simulink model "PE_V2_0"  (R2020b)
settings: Solver=VariableStepAuto  StartTime=0.0  StopTime=10.0  RelTol=1e-3
undefined symbols (not defined in the file): ZERO
libraries: hdlsllib x35, simulink x28, visionhdlutilities x12
(part 2 of 3)

== system PE_V2_0/2DConvPE1 V2.0/Subsystem2 ==
  In1 : Inport
  Bus Selector : BusSelector  OutputSignals=signal1,signal2,signal3,signal4,signal5,signal6,signal7,signal8,signal9,signal10,signal11,signal12,signal13,signal14,signal15
  Weight_Length : Outport
  Weight_Area : Outport  Port=2
  Weight_Width : Outport  Port=3
  Weight_Height : Outport  Port=4
  Feature_Length : Outport  Port=5
  Feature_Area : Outport  Port=6
  Feature_Width : Outport  Port=7
  Feature_Height : Outport  Port=8
  outFeature_Length : Outport  Port=9
  outFeature_Area : Outport  Port=10
  outFeature_Width : Outport  Port=11
  outFeature_Height : Outport  Port=12
  Conv_Step : Outport  Port=13
  Phase_in : Outport  Port=14
  Phase_out : Outport  Port=15
  wires:
  In1/1 -> Bus Selector/1
  Bus Selector/1 -> Weight_Length/1  "<signal1>"
  Bus Selector/2 -> Weight_Area/1  "<signal2>"
  Bus Selector/3 -> Weight_Width/1  "<signal3>"
  Bus Selector/4 -> Weight_Height/1  "<signal4>"
  Bus Selector/5 -> Feature_Length/1  "<signal5>"
  Bus Selector/6 -> Feature_Area/1  "<signal6>"
  Bus Selector/7 -> Feature_Width/1  "<signal7>"
  Bus Selector/8 -> Feature_Height/1  "<signal8>"
  Bus Selector/9 -> outFeature_Length/1  "<signal9>"
  Bus Selector/10 -> outFeature_Area/1  "<signal10>"
  Bus Selector/11 -> outFeature_Width/1  "<signal11>"
  Bus Selector/12 -> outFeature_Height/1  "<signal12>"
  Bus Selector/13 -> Conv_Step/1  "<signal13>"
  Bus Selector/14 -> Phase_in/1  "<signal14>"
  Bus Selector/15 -> Phase_out/1  "<signal15>"

== system PE_V2_0/2DCov PEV1.1/Adder Tree ==
  In1 : Inport
  In2 : Inport  Port=2
  In3 : Inport  Port=3
  In4 : Inport  Port=4
  In5 : Inport  Port=5
  In6 : Inport  Port=6
  In7 : Inport  Port=7
  In8 : Inport  Port=8
  In9 : Inport  Port=9
  validIn : Inport  Port=10
  Add{,1..6,10} (8 alike) : Sum
  Delay{1..9,35} (10 alike) : Delay  DelayLength=1
  Out1 : Outport
  validOut : Outport  Port=2
  wires:
  Add/1 -> Add4/1
  Add4/1 -> Add6/1
  Add10/1 -> Out1/1
  Add3/1 -> Add5/2
  Add2/1 -> Add5/1
  Add1/1 -> Add4/2
  Add6/1 -> Add10/1
  Add5/1 -> Add6/2
  Delay35/1 -> Add/1
  Delay1/1 -> Add/2
  Delay3/1 -> Add1/1
  Delay2/1 -> Add1/2
  Delay5/1 -> Add2/1
  Delay4/1 -> Add2/2
  Delay7/1 -> Add3/1
  Delay6/1 -> Add3/2
  In9/1 -> Delay8/1
  Delay8/1 -> Add10/2
  In8/1 -> Delay6/1
  In7/1 -> Delay7/1
  In6/1 -> Delay4/1
  In5/1 -> Delay5/1
  In4/1 -> Delay2/1
  In3/1 -> Delay3/1
  In2/1 -> Delay1/1
  In1/1 -> Delay35/1
  validIn/1 -> Delay9/1
  Delay9/1 -> validOut/1

== system PE_V2_0/2DCov PEV1.1/Address Logic ==
  note: W/R_Address_Gen
  In1 : Inport
  In2 : Inport  Port=2
  " " : Subsystem
  Add : Sum  Inputs=+-
  Compare To Constant : simulink/Logic and Bit Operations/Compare To Constant  relop===  const=0  OutDataTypeStr=boolean
  Constant : Constant  OutDataTypeStr=uint32
  Delay : Delay  DelayLength=1
  Logical Operator1 : Logic  AllPortsSameDT=off  OutDataTypeStr=boolean
  Logical Operator2 : Logic  Operator=NOT  AllPortsSameDT=off  OutDataTypeStr=boolean
  Relational Operator : RelationalOperator  OutDataTypeStr=boolean  RndMeth=Simplest
  Weight_Counter : hdlsllib/Sources/HDL Counter  CountType=Free running  CountInit=0  CountStep=1  CountMax=2^15  CountFromType=Initial value  CountFrom=0  CountResetPort=on  CountLoadPort=off  CountEnbPort=on  CountDirPort=off  CountDataType=Unsigned  CountWordLen=32  CountFracLen=0  CountSampTime=1
  Weight_Interation_Counter : hdlsllib/Sources/HDL Counter  CountType=Free running  CountInit=0  CountStep=1  CountMax=2^15  CountFromType=Initial value  CountFrom=0  CountResetPort=on  CountLoadPort=off  CountEnbPort=on  CountDirPort=off  CountDataType=Unsigned  CountWordLen=32  CountFracLen=0  CountSampTime=1
  W : Outport
  Write_en : Outport  Port=2
  R : Outport  Port=3
  wires:
  Weight_Counter/1 -> " "/1(In1), Relational Operator/1
  Compare To Constant/1 -> Write_en/1, " "/2(In2)
  Delay/1 -> Logical Operator1/2, Logical Operator2/1, Weight_Counter/2
  Weight_Interation_Counter/1 -> Compare To Constant/1
  Constant/1 -> Add/2
  Logical Operator2/1 -> Weight_Interation_Counter/1
  " "/1(W) -> W/1
  Logical Operator1/1 -> Weight_Counter/1
  Relational Operator/1 -> Weight_Interation_Counter/2, Logical Operator1/1
  Add/1 -> Relational Operator/2
  In1/1 -> Delay/1
  In2/1 -> Add/1
  " "/2(R) -> R/1

== system PE_V2_0/2DCov PEV1.1/LIne Buffer ==
  Stream_In : Inport
  Stream_Valid : Inport  Port=2
  Weight_Width : Inport  Port=3
  Feature_Area : Inport  Port=4
  Feature_Width : Inport  Port=5
  Feature_Height : Inport  Port=6
  Delay2 : Delay  DelayLength=1
  Line Buffer : Subsystem
  OutValidGen : Subsystem
  Terminator : Terminator
  pixel : Outport
  valid : Outport  Port=2
  wires:
  Feature_Area/1 -> Line Buffer/3(Feature_Area)
  Feature_Height/1 -> OutValidGen/3(Feature_Height)
  Line Buffer/3(shftEnable) -> Terminator/1
  Stream_In/1 -> Line Buffer/1(Stream_In)
  Line Buffer/1(pixel) -> Delay2/1
  Line Buffer/2(ctrl) -> OutValidGen/1(In1)
  Feature_Width/1 -> Line Buffer/4(Feature_Width)
  Stream_Valid/1 -> Line Buffer/2(Stream_Valid)
  Weight_Width/1 -> OutValidGen/2(Weight_Width)
  OutValidGen/1(valid) -> valid/1
  Delay2/1 -> pixel/1

== system PE_V2_0/2DCov PEV1.1/MaxPooling ==
  Stream_In : Inport
  Stream_Valid : Inport  Port=2
  ByPass : Inport  Port=3
  step : Inport  Port=4
  Window_Width : Inport  Port=5
  Feature_Area : Inport  Port=6
  Feature_Width : Inport  Port=7
  Feature_Height : Inport  Port=8
  Comparator : Subsystem
  Constant : Constant  Value=0  OutDataTypeStr=int32
  Delay{,1..6,36} (8 alike) : Delay  DelayLength=1
  Line Buffer1 : Subsystem
  OutValidGen : Subsystem
  Switch : Switch  Criteria=u2 > Threshold
  Switch1 : Switch  Criteria=u2 > Threshold
  Terminator1 : Terminator
  dataSwitch : Switch  Criteria=u2 > Threshold
  validSwitch : Switch  Criteria=u2 > Threshold
  window Selector : Subsystem
  outdata : Outport
  Valid : Outport  Port=2
  wires:
  window Selector/3(Out3) -> Delay3/1
  OutValidGen/1(Out1) -> window Selector/2(valid)
  Feature_Width/1 -> Line Buffer1/4(Feature_Width)
  Line Buffer1/3(shftEnable) -> Terminator1/1
  Window_Width/1 -> OutValidGen/2(Window_Width)
  window Selector/5(Valid) -> Delay5/1
  window Selector/1(Out1) -> Delay/1
  Line Buffer1/1(pixel) -> Delay2/1
  Line Buffer1/2(ctrl) -> OutValidGen/1(ctrl)
  window Selector/2(Out2) -> Delay6/1
  window Selector/4(Out4) -> Delay4/1
  Feature_Area/1 -> Line Buffer1/3(Feature_Area)
  Feature_Height/1 -> OutValidGen/3(Feature_Height)
  step/1 -> window Selector/3(step)
  Delay1/1 -> validSwitch/1, Switch1/3
  Comparator/1(Out1) -> dataSwitch/3
  Delay36/1 -> dataSwitch/1, Switch/3
  ByPass/1 -> validSwitch/2, dataSwitch/2, Switch1/2, Switch/2
  dataSwitch/1 -> outdata/1
  validSwitch/1 -> Valid/1
  Constant/1 -> Switch1/1, Switch/1
  Switch/1 -> Line Buffer1/1(Stream_In)
  Switch1/1 -> Line Buffer1/2(Stream_Valid)
  Comparator/2(outvalid) -> validSwitch/3
  Stream_In/1 -> Delay36/1
  Stream_Valid/1 -> Delay1/1
  Delay2/1 -> window Selector/1(pixel)
  Delay/1 -> Comparator/1(In1)
  Delay5/1 -> Comparator/5(Valid)
  Delay4/1 -> Comparator/4(In4)
  Delay3/1 -> Comparator/3(In3)
  Delay6/1 -> Comparator/2(In2)

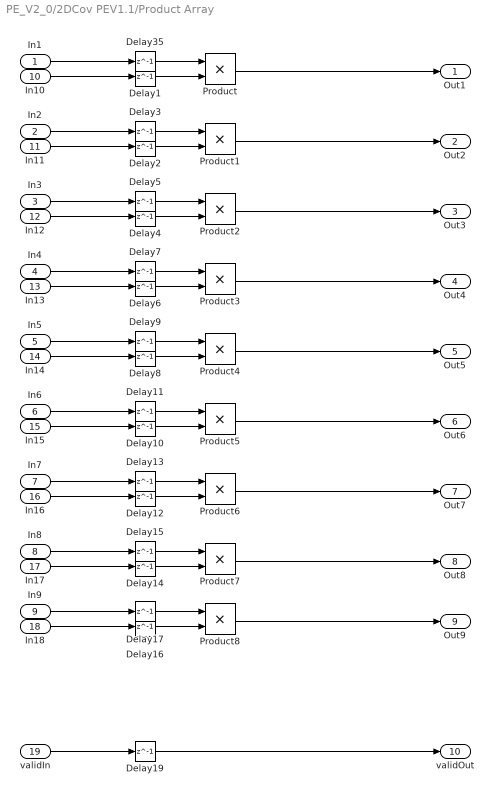
== system PE_V2_0/2DCov PEV1.1/Product Array ==
  In1 : Inport
  In2 : Inport  Port=2
  In3 : Inport  Port=3
  In4 : Inport  Port=4
  In5 : Inport  Port=5
  In6 : Inport  Port=6
  In7 : Inport  Port=7
  In8 : Inport  Port=8
  In9 : Inport  Port=9
  In10 : Inport  Port=10
  In11 : Inport  Port=11
  In12 : Inport  Port=12
  In13 : Inport  Port=13
  In14 : Inport  Port=14
  In15 : Inport  Port=15
  In16 : Inport  Port=16
  In17 : Inport  Port=17
  In18 : Inport  Port=18
  validIn : Inport  Port=19
  Delay{1..17,19,35} (19 alike) : Delay  DelayLength=1
  Product{,1..8} (9 alike) : Product
  Out1 : Outport
  Out2 : Outport  Port=2
  Out3 : Outport  Port=3
  Out4 : Outport  Port=4
  Out5 : Outport  Port=5
  Out6 : Outport  Port=6
  Out7 : Outport  Port=7
  Out8 : Outport  Port=8
  Out9 : Outport  Port=9
  validOut : Outport  Port=10
  wires:
  Product/1 -> Out1/1
  In4/1 -> Delay7/1
  Product4/1 -> Out5/1
  In8/1 -> Delay15/1
  In17/1 -> Delay14/1
  In9/1 -> Delay17/1
  In12/1 -> Delay4/1
  In7/1 -> Delay13/1
  In1/1 -> Delay35/1
  In13/1 -> Delay6/1
  Product1/1 -> Out2/1
  In16/1 -> Delay12/1
  In10/1 -> Delay1/1
  In14/1 -> Delay8/1
  In18/1 -> Delay16/1
  Product8/1 -> Out9/1
  Product7/1 -> Out8/1
  In6/1 -> Delay11/1
  In2/1 -> Delay3/1
  In11/1 -> Delay2/1
  In15/1 -> Delay10/1
  In5/1 -> Delay9/1
  In3/1 -> Delay5/1
  Product3/1 -> Out4/1
  Product2/1 -> Out3/1
  Product5/1 -> Out6/1
  Product6/1 -> Out7/1
  validIn/1 -> Delay19/1
  Delay1/1 -> Product/2
  Delay35/1 -> Product/1
  Delay3/1 -> Product1/1
  Delay2/1 -> Product1/2
  Delay5/1 -> Product2/1
  Delay4/1 -> Product2/2
  Delay7/1 -> Product3/1
  Delay6/1 -> Product3/2
  Delay8/1 -> Product4/2
  Delay9/1 -> Product4/1
  Delay11/1 -> Product5/1
  Delay10/1 -> Product5/2
  Delay13/1 -> Product6/1
  Delay12/1 -> Product6/2
  Delay14/1 -> Product7/2
  Delay15/1 -> Product7/1
  Delay17/1 -> Product8/1
  Delay16/1 -> Product8/2
  Delay19/1 -> validOut/1

== system PE_V2_0/2DCov PEV1.1/ReLU ==
  data_in : Inport
  validIn : Inport  Port=2
  byPass : Inport  Port=3
  Compare To Zero : simulink/Logic and Bit Operations/Compare To Zero  relop=>  OutDataTypeStr=boolean
  Constant : Constant  Value=0  OutDataTypeStr=int32
  Delay1 : Delay  DelayLength=1
  Delay36 : Delay  DelayLength=1
  Switch : Switch  Criteria=u2 > Threshold
  Switch1 : Switch  Criteria=u2 > Threshold
  data_ReLU : Outport
  valildOut : Outport  Port=2
  wires:
  Constant/1 -> Switch/3
  Delay36/1 -> Switch1/1, Switch/1, Compare To Zero/1
  Compare To Zero/1 -> Switch/2
  Switch/1 -> Switch1/3
  byPass/1 -> Switch1/2
  Switch1/1 -> data_ReLU/1
  Delay1/1 -> valildOut/1
  data_in/1 -> Delay36/1
  validIn/1 -> Delay1/1

== system PE_V2_0/2DCov PEV1.1/Subsystem ==
  In1 : Inport
  Bus Selector : BusSelector  OutputSignals=signal1,signal2
  pool_step : Outport
  pool_Width : Outport  Port=2
  wires:
  Bus Selector/2 -> pool_Width/1  "<signal2>"
  Bus Selector/1 -> pool_step/1  "<signal1>"
  In1/1 -> Bus Selector/1

== system PE_V2_0/2DCov PEV1.1/Subsystem2 ==
  In1 : Inport
  Bus Selector : BusSelector  OutputSignals=signal1,signal2,signal3,signal4,signal5,signal6,signal7,signal8,signal9,signal10,signal11,signal12,signal13,signal14,signal15
  Weight_Length : Outport
  Weight_Area : Outport  Port=2
  Weight_Width : Outport  Port=3
  Weight_Height : Outport  Port=4
  Feature_Length : Outport  Port=5
  Feature_Area : Outport  Port=6
  Feature_Width : Outport  Port=7
  Feature_Height : Outport  Port=8
  outFeature_Length : Outport  Port=9
  outFeature_Area : Outport  Port=10
  outFeature_Width : Outport  Port=11
  outFeature_Height : Outport  Port=12
  Conv_Step : Outport  Port=13
  inChannel : Outport  Port=14
  outChannel : Outport  Port=15
  wires:
  In1/1 -> Bus Selector/1
  Bus Selector/1 -> Weight_Length/1  "<signal1>"
  Bus Selector/2 -> Weight_Area/1  "<signal2>"
  Bus Selector/3 -> Weight_Width/1  "<signal3>"
  Bus Selector/4 -> Weight_Height/1  "<signal4>"
  Bus Selector/5 -> Feature_Length/1  "<signal5>"
  Bus Selector/6 -> Feature_Area/1  "<signal6>"
  Bus Selector/7 -> Feature_Width/1  "<signal7>"
  Bus Selector/8 -> Feature_Height/1  "<signal8>"
  Bus Selector/9 -> outFeature_Length/1  "<signal9>"
  Bus Selector/10 -> outFeature_Area/1  "<signal10>"
  Bus Selector/11 -> outFeature_Width/1  "<signal11>"
  Bus Selector/12 -> outFeature_Height/1  "<signal12>"
  Bus Selector/13 -> Conv_Step/1  "<signal13>"
  Bus Selector/14 -> inChannel/1  "<signal14>"
  Bus Selector/15 -> outChannel/1  "<signal15>"

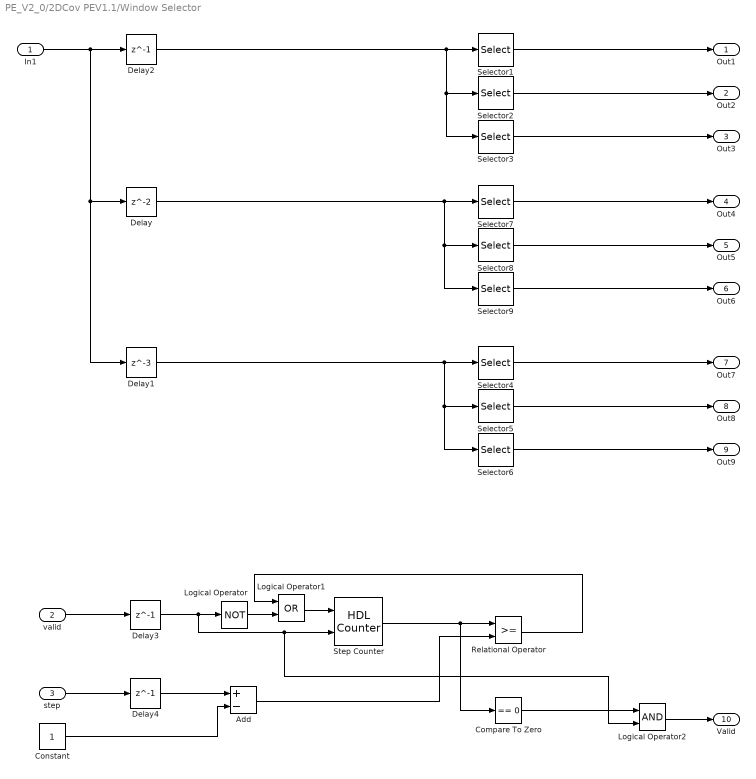
== system PE_V2_0/2DCov PEV1.1/Window Selector ==
  In1 : Inport
  valid : Inport  Port=2
  step : Inport  Port=3
  Add : Sum  Inputs=+-
  Compare To Zero : simulink/Logic and Bit Operations/Compare To Zero  relop===  OutDataTypeStr=boolean
  Constant : Constant  OutDataTypeStr=uint32
  Delay : Delay
  Delay1 : Delay  DelayLength=3
  Delay2 : Delay  DelayLength=1
  Delay3 : Delay  DelayLength=1
  Delay4 : Delay  DelayLength=1
  Logical Operator : Logic  Operator=NOT  AllPortsSameDT=off  OutDataTypeStr=boolean
  Logical Operator1 : Logic  Operator=OR  AllPortsSameDT=off  OutDataTypeStr=boolean
  Logical Operator2 : Logic  AllPortsSameDT=off  OutDataTypeStr=boolean
  Relational Operator : RelationalOperator  OutDataTypeStr=boolean  RndMeth=Nearest
  Selector1 : Selector  InputPortWidth=3  IndexOptions=Index vector (dialog)  Indices=[1]  OutputSizes=1
  Selector2 : Selector  InputPortWidth=3  IndexOptions=Index vector (dialog)  Indices=[2]  OutputSizes=1
  Selector3 : Selector  InputPortWidth=3  IndexOptions=Index vector (dialog)  Indices=[3]  OutputSizes=1
  Selector4 : Selector  InputPortWidth=3  IndexOptions=Index vector (dialog)  Indices=[1]  OutputSizes=1
  Selector5 : Selector  InputPortWidth=3  IndexOptions=Index vector (dialog)  Indices=[2]  OutputSizes=1
  Selector6 : Selector  InputPortWidth=3  IndexOptions=Index vector (dialog)  Indices=[3]  OutputSizes=1
  Selector7 : Selector  InputPortWidth=3  IndexOptions=Index vector (dialog)  Indices=[1]  OutputSizes=1
  Selector8 : Selector  InputPortWidth=3  IndexOptions=Index vector (dialog)  Indices=[2]  OutputSizes=1
  Selector9 : Selector  InputPortWidth=3  IndexOptions=Index vector (dialog)  Indices=[3]  OutputSizes=1
  Step Counter : hdlsllib/Sources/HDL Counter  CountType=Free running  CountInit=0  CountStep=1  CountMax=2^15  CountFromType=Initial value  CountFrom=0  CountResetPort=on  CountLoadPort=off  CountEnbPort=on  CountDirPort=off  CountDataType=Unsigned  CountWordLen=32  CountFracLen=0  CountSampTime=1
  Out1 : Outport
  Out2 : Outport  Port=2
  Out3 : Outport  Port=3
  Out4 : Outport  Port=4
  Out5 : Outport  Port=5
  Out6 : Outport  Port=6
  Out7 : Outport  Port=7
  Out8 : Outport  Port=8
  Out9 : Outport  Port=9
  Valid : Outport  Port=10
  wires:
  Selector2/1 -> Out2/1
  In1/1 -> Delay2/1, Delay1/1, Delay/1
  Selector1/1 -> Out1/1
  Selector3/1 -> Out3/1
  Selector8/1 -> Out5/1
  Selector9/1 -> Out6/1
  Selector7/1 -> Out4/1
  Delay/1 -> Selector9/1, Selector8/1, Selector7/1
  Selector5/1 -> Out8/1
  Selector6/1 -> Out9/1
  Selector4/1 -> Out7/1
  Delay1/1 -> Selector6/1, Selector5/1, Selector4/1
  Relational Operator/1 -> Logical Operator1/1
  Constant/1 -> Add/2
  Logical Operator2/1 -> Valid/1
  Compare To Zero/1 -> Logical Operator2/1
  Logical Operator1/1 -> Step Counter/1
  Logical Operator/1 -> Logical Operator1/2
  Delay4/1 -> Add/1
  Step Counter/1 -> Compare To Zero/1, Relational Operator/1
  Delay3/1 -> Logical Operator2/2, Step Counter/2, Logical Operator/1
  Add/1 -> Relational Operator/2
  Delay2/1 -> Selector3/1, Selector2/1, Selector1/1
  valid/1 -> Delay3/1
  step/1 -> Delay4/1

== system PE_V2_0/2DConvPE1 V1.5/FUNCTION/Adder Tree ==
  In1 : Inport
  In2 : Inport  Port=2
  In3 : Inport  Port=3
  In4 : Inport  Port=4
  In5 : Inport  Port=5
  In6 : Inport  Port=6
  In7 : Inport  Port=7
  In8 : Inport  Port=8
  In9 : Inport  Port=9
  validIn : Inport  Port=10
  Add{,1..6,10} (8 alike) : Sum
  Delay{1..9,35} (10 alike) : Delay  DelayLength=1
  dataOut : Outport
  validOut : Outport  Port=2
  wires:
  Add/1 -> Add4/1
  Add4/1 -> Add6/1
  Add10/1 -> dataOut/1
  Add3/1 -> Add5/2
  Add2/1 -> Add5/1
  Add1/1 -> Add4/2
  Add6/1 -> Add10/1
  Add5/1 -> Add6/2
  Delay35/1 -> Add/1
  Delay1/1 -> Add/2
  Delay3/1 -> Add1/1
  Delay2/1 -> Add1/2
  Delay5/1 -> Add2/1
  Delay4/1 -> Add2/2
  Delay7/1 -> Add3/1
  Delay6/1 -> Add3/2
  In9/1 -> Delay8/1
  Delay8/1 -> Add10/2
  In8/1 -> Delay6/1
  In7/1 -> Delay7/1
  In6/1 -> Delay4/1
  In5/1 -> Delay5/1
  In4/1 -> Delay2/1
  In3/1 -> Delay3/1
  In2/1 -> Delay1/1
  In1/1 -> Delay35/1
  validIn/1 -> Delay9/1
  Delay9/1 -> validOut/1

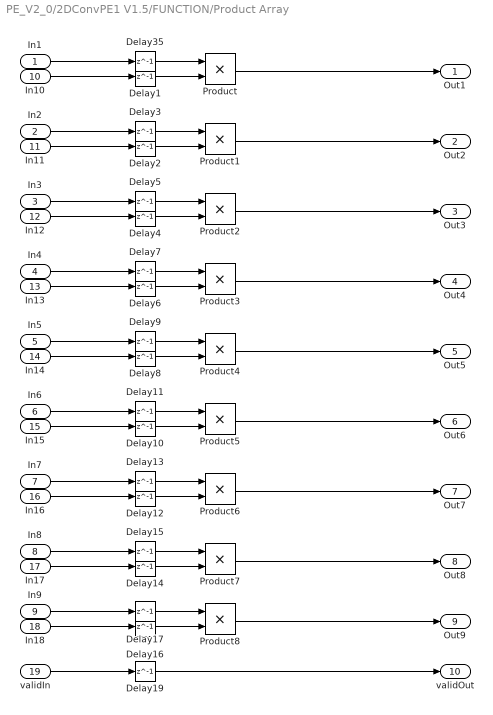
== system PE_V2_0/2DConvPE1 V1.5/FUNCTION/Product Array ==
  In1 : Inport
  In2 : Inport  Port=2
  In3 : Inport  Port=3
  In4 : Inport  Port=4
  In5 : Inport  Port=5
  In6 : Inport  Port=6
  In7 : Inport  Port=7
  In8 : Inport  Port=8
  In9 : Inport  Port=9
  In10 : Inport  Port=10
  In11 : Inport  Port=11
  In12 : Inport  Port=12
  In13 : Inport  Port=13
  In14 : Inport  Port=14
  In15 : Inport  Port=15
  In16 : Inport  Port=16
  In17 : Inport  Port=17
  In18 : Inport  Port=18
  validIn : Inport  Port=19
  Delay{1..17,19,35} (19 alike) : Delay  DelayLength=1
  Product{,1..8} (9 alike) : Product
  Out1 : Outport
  Out2 : Outport  Port=2
  Out3 : Outport  Port=3
  Out4 : Outport  Port=4
  Out5 : Outport  Port=5
  Out6 : Outport  Port=6
  Out7 : Outport  Port=7
  Out8 : Outport  Port=8
  Out9 : Outport  Port=9
  validOut : Outport  Port=10
  wires:
  Product/1 -> Out1/1
  In4/1 -> Delay7/1
  Product4/1 -> Out5/1
  In8/1 -> Delay15/1
  In17/1 -> Delay14/1
  In9/1 -> Delay17/1
  In12/1 -> Delay4/1
  In7/1 -> Delay13/1
  In1/1 -> Delay35/1
  In13/1 -> Delay6/1
  Product1/1 -> Out2/1
  In16/1 -> Delay12/1
  In10/1 -> Delay1/1
  In14/1 -> Delay8/1
  In18/1 -> Delay16/1
  Product8/1 -> Out9/1
  Product7/1 -> Out8/1
  In6/1 -> Delay11/1
  In2/1 -> Delay3/1
  In11/1 -> Delay2/1
  In15/1 -> Delay10/1
  In5/1 -> Delay9/1
  In3/1 -> Delay5/1
  Product3/1 -> Out4/1
  Product2/1 -> Out3/1
  Product5/1 -> Out6/1
  Product6/1 -> Out7/1
  validIn/1 -> Delay19/1
  Delay1/1 -> Product/2
  Delay35/1 -> Product/1
  Delay3/1 -> Product1/1
  Delay2/1 -> Product1/2
  Delay5/1 -> Product2/1
  Delay4/1 -> Product2/2
  Delay7/1 -> Product3/1
  Delay6/1 -> Product3/2
  Delay8/1 -> Product4/2
  Delay9/1 -> Product4/1
  Delay11/1 -> Product5/1
  Delay10/1 -> Product5/2
  Delay13/1 -> Product6/1
  Delay12/1 -> Product6/2
  Delay14/1 -> Product7/2
  Delay15/1 -> Product7/1
  Delay17/1 -> Product8/1
  Delay16/1 -> Product8/2
  Delay19/1 -> validOut/1

== system PE_V2_0/2DConvPE1 V1.5/FUNCTION/Subsystem1 ==
  weight_data_valid : Inport
  weight_data : Inport  Port=2
  Stream_In : Inport  Port=3
  Stream_Valid : Inport  Port=4
  Weight_Width : Inport  Port=5
  Feature_Area : Inport  Port=6
  Feature_Width : Inport  Port=7
  Feature_Height : Inport  Port=8
  stride : Inport  Port=9
  Delay4 : Delay
  Delay5 : Delay
  LIne Buffer : Subsystem
      settings: PortSchema="{\"entries\":[{\"content\":{\"sides\":[{\"content\":{\"connectorIds\":[\"In1\",\"In2\"]},\"type\":\"ConnectorPlacement.EquallySpacedRectSide\",\"uuid\":\"a250c848-7a40-462c-bfcf-0ff48046d99d\"},{\"content\":{\"connectorIds\":[\"Out1\",\"Out2\"],\"side\":\"RIGHT\"},\"type\":\"ConnectorPlacement.EquallySpacedRectSide\",\"uuid\":\"81aecf2d-6bfb-4d40-80c7-cfb89c921406\"},{\"content\":{\"connectorIds\":[],\"side\":\"TOP\"},\"type\":\"ConnectorPlacement.EquallySpacedRectSide\",\"uuid\":\"288ccc7a-b219-4526-a408-3d8b1082f4b0\"},{\"content\":{\"connectorIds\":[\"In3\",\"In4\",\"In5\",\"In6\"],\"side\":\"BOTTOM\"},\"type\":\"ConnectorPlacement.EquallySpacedRectSide\",\"uuid\":\"5d9529f5-ee70-4412-83ca-b280a2219284\"},{\"content\":{\"connectorIds\":[],\"side\":\"HIDDEN\"},\"type\":\"ConnectorPlacement.EquallySpacedRectSide\",\"uuid\":\"3d06d450-49b0-49ba-a273-690d97c3e8e1\"}]},\"type\":\"ConnectorPlacement.EquallySpacedConnector\",\"uuid\":\"b82e05d1-4695-4e04-9663-17698b30471b\"}],\"packageUris\":[\"http://schema.mathworks.com/mf0/Connector/R2020b\"],\"version\":\"1.0\"}"
  Window Selector : Subsystem
      settings: PortSchema="{\"entries\":[{\"content\":{\"sides\":[{\"content\":{\"connectorIds\":[\"In1\",\"In2\"]},\"type\":\"ConnectorPlacement.EquallySpacedRectSide\",\"uuid\":\"2f98ee57-d732-418e-86bd-7acbaf2524e0\"},{\"content\":{\"connectorIds\":[\"Out1\",\"Out2\",\"Out3\",\"Out4\",\"Out5\",\"Out6\",\"Out7\",\"Out8\",\"Out9\",\"Out10\"],\"side\":\"RIGHT\"},\"type\":\"ConnectorPlacement.EquallySpacedRectSide\",\"uuid\":\"287ad403-178f-48f1-9791-2ccad363e9c6\"},{\"content\":{\"connectorIds\":[],\"side\":\"TOP\"},\"type\":\"ConnectorPlacement.EquallySpacedRectSide\",\"uuid\":\"a860ecae-5cde-45ef-a487-fdb4fb7390aa\"},{\"content\":{\"connectorIds\":[\"In3\"],\"side\":\"BOTTOM\"},\"type\":\"ConnectorPlacement.EquallySpacedRectSide\",\"uuid\":\"925435f5-0fb8-4a67-9f76-fe99b5b92634\"},{\"content\":{\"connectorIds\":[],\"side\":\"HIDDEN\"},\"type\":\"ConnectorPlacement.EquallySpacedRectSide\",\"uuid\":\"e6f3edac-a41a-4276-8ae6-cd8be9b02af9\"}]},\"type\":\"ConnectorPlacement.EquallySpacedConnector\",\"uuid\":\"0e32a9d0-da82-46c8-ab50-9de41c4380a9\"}],\"packageUris\":[\"http://schema.mathworks.com/mf0/Connector/R2020b\"],\"version\":\"1.0\"}"
  weight_register : Subsystem
  Out1 : Outport
  Out2 : Outport  Port=2
  Out3 : Outport  Port=3
  Out4 : Outport  Port=4
  Out5 : Outport  Port=5
  Out6 : Outport  Port=6
  Out7 : Outport  Port=7
  Out8 : Outport  Port=8
  Out9 : Outport  Port=9
  Out10 : Outport  Port=10
  Out11 : Outport  Port=11
  Out12 : Outport  Port=12
  Out13 : Outport  Port=13
  Out14 : Outport  Port=14
  Out15 : Outport  Port=15
  Out16 : Outport  Port=16
  Out17 : Outport  Port=17
  Out18 : Outport  Port=18
  Valid : Outport  Port=19
  wires:
  weight_register/4(Out5) -> Out4/1
  LIne Buffer/2(valid) -> Window Selector/2(valid)
  Window Selector/8(Out8) -> Out17/1
  weight_register/6(Out7) -> Out6/1
  weight_data/1 -> Delay4/1
  weight_register/9(Out1) -> Out9/1
  weight_data_valid/1 -> Delay5/1
  weight_register/2(Out3) -> Out2/1
  stride/1 -> Window Selector/3(stride)
  Feature_Height/1 -> LIne Buffer/6(Feature_Height)
  Delay4/1 -> weight_register/1(In1)
  LIne Buffer/1(pixel) -> Window Selector/1(In1)
  Stream_In/1 -> LIne Buffer/1(Stream_In)
  Delay5/1 -> weight_register/Enable
  Weight_Width/1 -> LIne Buffer/3(Weight_Width)
  weight_register/5(Out6) -> Out5/1
  weight_register/1(Out2) -> Out1/1
  Window Selector/4(Out4) -> Out13/1
  Feature_Width/1 -> LIne Buffer/5(Feature_Width)
  Window Selector/2(Out2) -> Out11/1
  weight_register/3(Out4) -> Out3/1
  Feature_Area/1 -> LIne Buffer/4(Feature_Area)
  Stream_Valid/1 -> LIne Buffer/2(Stream_Valid)
  weight_register/8(Out9) -> Out8/1
  weight_register/7(Out8) -> Out7/1
  Window Selector/5(Out5) -> Out14/1
  Window Selector/3(Out3) -> Out12/1
  Window Selector/9(Out9) -> Out18/1
  Window Selector/6(Out6) -> Out15/1
  Window Selector/7(Out7) -> Out16/1
  Window Selector/1(Out1) -> Out10/1
  Window Selector/10(Valid) -> Valid/1

== system PE_V2_0/2DConvPE1 V1.5/MaxPooling/Comparator ==
  In1 : Inport
  In2 : Inport  Port=2
  In3 : Inport  Port=3
  In4 : Inport  Port=4
  Valid : Inport  Port=5
  Delay{,1..4} (5 alike) : Delay  DelayLength=1
  Relational Operator : RelationalOperator  Operator=>  OutDataTypeStr=boolean  RndMeth=Nearest
  Relational Operator1 : RelationalOperator  Operator=>  OutDataTypeStr=boolean  RndMeth=Nearest
  Relational Operator2 : RelationalOperator  Operator=>  OutDataTypeStr=boolean  RndMeth=Nearest
  Switch : Switch  Criteria=u2 > Threshold
  Switch1 : Switch  Criteria=u2 > Threshold
  Switch2 : Switch  Criteria=u2 > Threshold
  Out1 : Outport
  outvalid : Outport  Port=2
  wires:
  Switch1/1 -> Relational Operator2/2, Switch2/3
  Switch/1 -> Switch2/1, Relational Operator2/1
  Delay/1 -> Switch/1, Relational Operator/1
  Relational Operator/1 -> Switch/2
  Relational Operator1/1 -> Switch1/2
  In2/1 -> Delay1/1
  In3/1 -> Delay2/1
  Relational Operator2/1 -> Switch2/2
  In4/1 -> Delay3/1
  Switch2/1 -> Out1/1
  Valid/1 -> Delay4/1
  Delay1/1 -> Relational Operator/2, Switch/3
  Delay2/1 -> Switch1/1, Relational Operator1/1
  In1/1 -> Delay/1
  Delay3/1 -> Relational Operator1/2, Switch1/3
  Delay4/1 -> outvalid/1

== system PE_V2_0/2DConvPE1 V1.5/MaxPooling/Line Buffer1 ==
  Stream_In : Inport
  Stream_Valid : Inport  Port=2
  Feature_Area : Inport  Port=3
  Feature_Width : Inport  Port=4
  CtrlGen : Subsystem
  Line Buffer : visionhdlutilities/Line Buffer  NeighborhoodSize=[2 1]  PaddingMethod=Constant  PaddingValue=0  LineBufferSize=128  SimulateUsing=Code generation
      settings: SourceProductBaseCode=VT
  pixel : Outport
  ctrl : Outport  Port=2
  shftEnable : Outport  Port=3
  wires:
  Feature_Area/1 -> CtrlGen/3(Feature_Area)
  Line Buffer/2 -> ctrl/1
  CtrlGen/1(StreamOut) -> Line Buffer/1
  Feature_Width/1 -> CtrlGen/4(Feature_Width)
  Stream_In/1 -> CtrlGen/1(Stream_In)
  CtrlGen/2(Ctrl) -> Line Buffer/2
  Stream_Valid/1 -> CtrlGen/2(Stream_Valid)
  Line Buffer/3 -> shftEnable/1
  Line Buffer/1 -> pixel/1

== system PE_V2_0/2DConvPE1 V1.5/MaxPooling/OutValidGen ==
  ctrl : Inport
  Window_Width : Inport  Port=2
  Feature_Height : Inport  Port=3
  Compare To Constant : simulink/Logic and Bit Operations/Compare To Constant  Commented=on  relop=>  const=0  OutDataTypeStr=boolean
  Constant : Constant  OutDataTypeStr=uint32  SampleTime=-1
  Delay36 : Delay  DelayLength=1
  Logical Operator1 : Logic  Operator=NOT  AllPortsSameDT=off  OutDataTypeStr=boolean
  Logical Operator3 : Logic  Inputs=3  AllPortsSameDT=off  OutDataTypeStr=boolean
  Logical Operator4 : Logic  Operator=NOT  AllPortsSameDT=off  OutDataTypeStr=boolean
  Logical Operator5 : Logic  Operator=OR  AllPortsSameDT=off  OutDataTypeStr=boolean
  Logical Operator6 : Logic  Operator=NOT  Inputs=3  AllPortsSameDT=off  OutDataTypeStr=boolean
  Minus1 : Sum  Inputs=+-
  Minus2 : Sum  Inputs=+-
  NumRow_Counter : hdlsllib/Sources/HDL Counter  CountType=Free running  CountInit=0  CountStep=1  CountMax=2^15  CountFromType=Initial value  CountFrom=0  CountResetPort=on  CountLoadPort=off  CountEnbPort=on  CountDirPort=off  CountDataType=Unsigned  CountWordLen=32  CountFracLen=0  CountSampTime=1
  Pixel Control Bus Selector : BusSelector  OutputSignals=hStart,hEnd,vStart,vEnd,valid
  Relational Operator1 : RelationalOperator  Operator=<  OutDataTypeStr=boolean  RndMeth=Nearest
  Relational Operator2 : RelationalOperator  Operator=<=  OutDataTypeStr=boolean  RndMeth=Nearest
  Row_Counter : hdlsllib/Sources/HDL Counter  CountType=Free running  CountInit=0  CountStep=1  CountMax=2^15  CountFromType=Initial value  CountFrom=0  CountResetPort=on  CountLoadPort=off  CountEnbPort=on  CountDirPort=off  CountDataType=Unsigned  CountWordLen=32  CountFracLen=0  CountSampTime=1
  Terminator1 : Terminator
  Out1 : Outport
  wires:
  NumRow_Counter/1 -> Relational Operator2/2, Compare To Constant/1
  Pixel Control Bus Selector/1 -> NumRow_Counter/2  "<hStart>"
  Minus2/1 -> Relational Operator2/1
  Relational Operator1/1 -> Logical Operator4/1
  Pixel Control Bus Selector/3 -> Logical Operator5/1  "<vStart>"
  Feature_Height/1 -> Minus2/1
  Minus1/1 -> Relational Operator1/2
  Row_Counter/1 -> Relational Operator1/1
  Pixel Control Bus Selector/5 -> Row_Counter/2, Logical Operator1/1, Logical Operator3/2  "<valid>"
  Window_Width/1 -> Minus1/1
  Pixel Control Bus Selector/2 -> Terminator1/1  "<hEnd>"
  Delay36/1 -> Pixel Control Bus Selector/1
  Constant/1 -> Minus1/2, Minus2/2
  Logical Operator6/1 -> Logical Operator3/1
  Logical Operator5/1 -> NumRow_Counter/1
  Pixel Control Bus Selector/4 -> Logical Operator5/2  "<vEnd>"
  Relational Operator2/1 -> Logical Operator6/1
  Logical Operator1/1 -> Row_Counter/1
  Logical Operator4/1 -> Logical Operator3/3
  Logical Operator3/1 -> Out1/1
  ctrl/1 -> Delay36/1

== system PE_V2_0/2DConvPE1 V1.5/MaxPooling/window Selector ==
  pixel : Inport
  valid : Inport  Port=2
  step : Inport  Port=3
  Add : Sum  Inputs=+-
  Compare To Zero : simulink/Logic and Bit Operations/Compare To Zero  relop===  OutDataTypeStr=boolean
  Constant : Constant  OutDataTypeStr=uint32
  Delay : Delay
  Delay1 : Delay  DelayLength=1
  Delay36 : Delay  DelayLength=1
  Logical Operator : Logic  Operator=NOT  AllPortsSameDT=off  OutDataTypeStr=boolean
  Logical Operator1 : Logic  Operator=OR  AllPortsSameDT=off  OutDataTypeStr=boolean
  Logical Operator2 : Logic  AllPortsSameDT=off  OutDataTypeStr=boolean
  Relational Operator : RelationalOperator  OutDataTypeStr=boolean  RndMeth=Nearest
  Selector1 : Selector  InputPortWidth=2  IndexOptions=Index vector (dialog)  Indices=[1]  OutputSizes=1
  Selector2 : Selector  InputPortWidth=2  IndexOptions=Index vector (dialog)  Indices=[2]  OutputSizes=1
  Selector3 : Selector  InputPortWidth=2  IndexOptions=Index vector (dialog)  Indices=[1]  OutputSizes=1
  Selector4 : Selector  InputPortWidth=2  IndexOptions=Index vector (dialog)  Indices=[2]  OutputSizes=1
  Step Counter : hdlsllib/Sources/HDL Counter  CountType=Free running  CountInit=0  CountStep=1  CountMax=2^15  CountFromType=Initial value  CountFrom=0  CountResetPort=on  CountLoadPort=off  CountEnbPort=on  CountDirPort=off  CountDataType=Unsigned  CountWordLen=32  CountFracLen=0  CountSampTime=1
  Out1 : Outport
  Out2 : Outport  Port=2
  Out3 : Outport  Port=3
  Out4 : Outport  Port=4
  Valid : Outport  Port=5
  wires:
  Selector2/1 -> Out2/1
  Delay/1 -> Selector4/1, Selector3/1
  Selector3/1 -> Out3/1
  Selector1/1 -> Out1/1
  Selector4/1 -> Out4/1
  pixel/1 -> Delay36/1, Delay/1
  Step Counter/1 -> Compare To Zero/1, Relational Operator/1
  Delay1/1 -> Logical Operator2/2, Step Counter/2, Logical Operator/1
  Logical Operator/1 -> Logical Operator1/2
  step/1 -> Add/1
  Constant/1 -> Add/2
  Add/1 -> Relational Operator/2
  Relational Operator/1 -> Logical Operator1/1
  Logical Operator1/1 -> Step Counter/1
  Compare To Zero/1 -> Logical Operator2/1
  Logical Operator2/1 -> Valid/1
  Delay36/1 -> Selector2/1, Selector1/1
  valid/1 -> Delay1/1

== system PE_V2_0/2DConvPE1 V2.0/Line Buffer/LIne Buffer ==
  Stream_In : Inport
  Stream_Valid : Inport  Port=2
  Weight_Width : Inport  Port=3
  Feature_Area : Inport  Port=4
  Feature_Width : Inport  Port=5
  Feature_Height : Inport  Port=6
  Delay2 : Delay  DelayLength=1
  Line Buffer : Subsystem
  OutValidGen : Subsystem
  Terminator : Terminator
  pixel : Outport
  valid : Outport  Port=2
  wires:
  Feature_Area/1 -> Line Buffer/3(Feature_Area)
  Feature_Height/1 -> OutValidGen/3(Feature_Height)
  Line Buffer/3(shftEnable) -> Terminator/1
  Stream_In/1 -> Line Buffer/1(Stream_In)
  Line Buffer/1(pixel) -> Delay2/1
  Line Buffer/2(ctrl) -> OutValidGen/1(In1)
  Feature_Width/1 -> Line Buffer/4(Feature_Width)
  Stream_Valid/1 -> Line Buffer/2(Stream_Valid)
  Weight_Width/1 -> OutValidGen/2(Weight_Width)
  OutValidGen/1(valid) -> valid/1
  Delay2/1 -> pixel/1

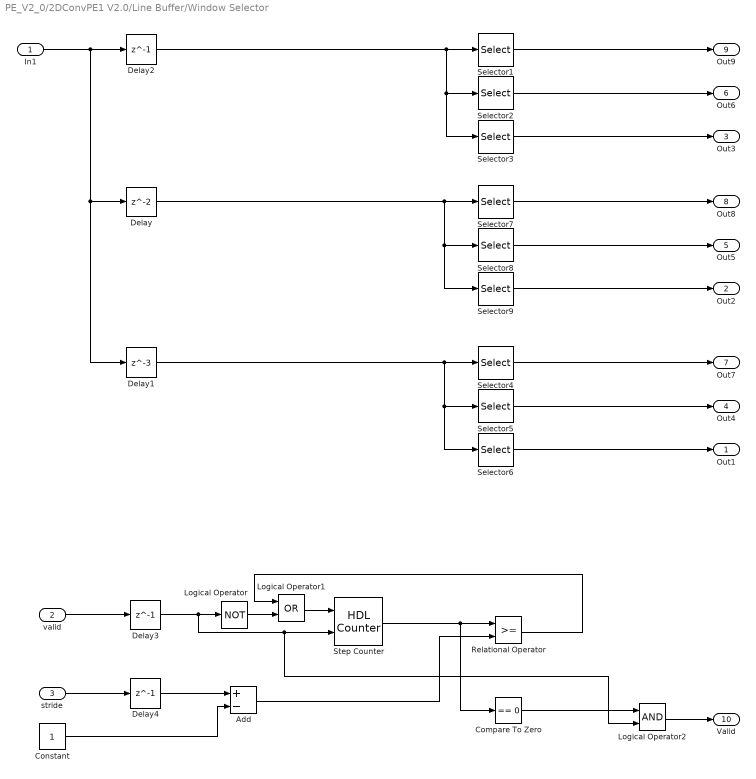
== system PE_V2_0/2DConvPE1 V2.0/Line Buffer/Window Selector ==
  In1 : Inport
  valid : Inport  Port=2
  stride : Inport  Port=3
  Add : Sum  Inputs=+-
  Compare To Zero : simulink/Logic and Bit Operations/Compare To Zero  relop===  OutDataTypeStr=boolean
  Constant : Constant  OutDataTypeStr=uint32
  Delay : Delay
  Delay1 : Delay  DelayLength=3
  Delay2 : Delay  DelayLength=1
  Delay3 : Delay  DelayLength=1
  Delay4 : Delay  DelayLength=1
  Logical Operator : Logic  Operator=NOT  AllPortsSameDT=off  OutDataTypeStr=boolean
  Logical Operator1 : Logic  Operator=OR  AllPortsSameDT=off  OutDataTypeStr=boolean
  Logical Operator2 : Logic  AllPortsSameDT=off  OutDataTypeStr=boolean
  Relational Operator : RelationalOperator  OutDataTypeStr=boolean  RndMeth=Nearest
  Selector1 : Selector  InputPortWidth=3  IndexOptions=Index vector (dialog)  Indices=[1]  OutputSizes=1
  Selector2 : Selector  InputPortWidth=3  IndexOptions=Index vector (dialog)  Indices=[2]  OutputSizes=1
  Selector3 : Selector  InputPortWidth=3  IndexOptions=Index vector (dialog)  Indices=[3]  OutputSizes=1
  Selector4 : Selector  InputPortWidth=3  IndexOptions=Index vector (dialog)  Indices=[1]  OutputSizes=1
  Selector5 : Selector  InputPortWidth=3  IndexOptions=Index vector (dialog)  Indices=[2]  OutputSizes=1
  Selector6 : Selector  InputPortWidth=3  IndexOptions=Index vector (dialog)  Indices=[3]  OutputSizes=1
  Selector7 : Selector  InputPortWidth=3  IndexOptions=Index vector (dialog)  Indices=[1]  OutputSizes=1
  Selector8 : Selector  InputPortWidth=3  IndexOptions=Index vector (dialog)  Indices=[2]  OutputSizes=1
  Selector9 : Selector  InputPortWidth=3  IndexOptions=Index vector (dialog)  Indices=[3]  OutputSizes=1
  Step Counter : hdlsllib/Sources/HDL Counter  CountType=Free running  CountInit=0  CountStep=1  CountMax=2^15  CountFromType=Initial value  CountFrom=0  CountResetPort=on  CountLoadPort=off  CountEnbPort=on  CountDirPort=off  CountDataType=Unsigned  CountWordLen=32  CountFracLen=0  CountSampTime=1
  Out1 : Outport
  Out2 : Outport  Port=2
  Out3 : Outport  Port=3
  Out4 : Outport  Port=4
  Out5 : Outport  Port=5
  Out6 : Outport  Port=6
  Out7 : Outport  Port=7
  Out8 : Outport  Port=8
  Out9 : Outport  Port=9
  Valid : Outport  Port=10
  wires:
  In1/1 -> Delay2/1, Delay1/1, Delay/1
  Selector9/1 -> Out2/1
  Delay/1 -> Selector9/1, Selector8/1, Selector7/1
  Selector5/1 -> Out4/1
  Selector6/1 -> Out1/1
  Selector4/1 -> Out7/1
  Delay1/1 -> Selector6/1, Selector5/1, Selector4/1
  Relational Operator/1 -> Logical Operator1/1
  Constant/1 -> Add/2
  Logical Operator2/1 -> Valid/1
  Compare To Zero/1 -> Logical Operator2/1
  Logical Operator1/1 -> Step Counter/1
  Logical Operator/1 -> Logical Operator1/2
  Delay4/1 -> Add/1
  Step Counter/1 -> Compare To Zero/1, Relational Operator/1
  Delay3/1 -> Logical Operator2/2, Step Counter/2, Logical Operator/1
  Add/1 -> Relational Operator/2
  Delay2/1 -> Selector3/1, Selector2/1, Selector1/1
  valid/1 -> Delay3/1
  stride/1 -> Delay4/1
  Selector8/1 -> Out5/1
  Selector7/1 -> Out8/1
  Selector3/1 -> Out3/1
  Selector2/1 -> Out6/1
  Selector1/1 -> Out9/1

== system PE_V2_0/2DConvPE1 V2.0/Line Buffer/weight_register ==
  In1 : Inport
  Enable : EnablePort
  Delay{1,3..8,40} (8 alike) : Delay  DelayLength=1
  Out2 : Outport
  Out3 : Outport  Port=2
  Out4 : Outport  Port=3
  Out5 : Outport  Port=4
  Out6 : Outport  Port=5
  Out7 : Outport  Port=6
  Out8 : Outport  Port=7
  Out9 : Outport  Port=8
  Out1 : Outport  Port=9
  wires:
  Delay40/1 -> Delay7/1, Out9/1
  In1/1 -> Out1/1, Delay40/1
  Delay7/1 -> Out8/1, Delay1/1
  Delay1/1 -> Out7/1, Delay5/1
  Delay5/1 -> Out6/1, Delay8/1
  Delay8/1 -> Out5/1, Delay6/1
  Delay6/1 -> Out4/1, Delay4/1
  Delay4/1 -> Out3/1, Delay3/1
  Delay3/1 -> Out2/1

== system PE_V2_0/2DConvPE1 V2.0/MaxPooling/Comparator ==
  In1 : Inport
  In2 : Inport  Port=2
  In3 : Inport  Port=3
  In4 : Inport  Port=4
  Valid : Inport  Port=5
  Delay{,1..4} (5 alike) : Delay  DelayLength=1
  Relational Operator : RelationalOperator  Operator=>  OutDataTypeStr=boolean  RndMeth=Nearest
  Relational Operator1 : RelationalOperator  Operator=>  OutDataTypeStr=boolean  RndMeth=Nearest
  Relational Operator2 : RelationalOperator  Operator=>  OutDataTypeStr=boolean  RndMeth=Nearest
  Switch : Switch  Criteria=u2 > Threshold
  Switch1 : Switch  Criteria=u2 > Threshold
  Switch2 : Switch  Criteria=u2 > Threshold
  Out1 : Outport
  outvalid : Outport  Port=2
  wires:
  Switch1/1 -> Relational Operator2/2, Switch2/3
  Switch/1 -> Switch2/1, Relational Operator2/1
  Delay/1 -> Switch/1, Relational Operator/1
  Relational Operator/1 -> Switch/2
  Relational Operator1/1 -> Switch1/2
  In2/1 -> Delay1/1
  In3/1 -> Delay2/1
  Relational Operator2/1 -> Switch2/2
  In4/1 -> Delay3/1
  Switch2/1 -> Out1/1
  Valid/1 -> Delay4/1
  Delay1/1 -> Relational Operator/2, Switch/3
  Delay2/1 -> Switch1/1, Relational Operator1/1
  In1/1 -> Delay/1
  Delay3/1 -> Relational Operator1/2, Switch1/3
  Delay4/1 -> outvalid/1

== system PE_V2_0/2DConvPE1 V2.0/MaxPooling/Line Buffer1 ==
  Stream_In : Inport
  Stream_Valid : Inport  Port=2
  Feature_Area : Inport  Port=3
  Feature_Width : Inport  Port=4
  CtrlGen : Subsystem
  Line Buffer : visionhdlutilities/Line Buffer  NeighborhoodSize=[2 1]  PaddingMethod=Constant  PaddingValue=0  LineBufferSize=128  SimulateUsing=Code generation
      settings: SourceProductBaseCode=VT
  pixel : Outport
  ctrl : Outport  Port=2
  shftEnable : Outport  Port=3
  wires:
  Feature_Area/1 -> CtrlGen/3(Feature_Area)
  Line Buffer/2 -> ctrl/1
  CtrlGen/1(StreamOut) -> Line Buffer/1
  Feature_Width/1 -> CtrlGen/4(Feature_Width)
  Stream_In/1 -> CtrlGen/1(Stream_In)
  CtrlGen/2(Ctrl) -> Line Buffer/2
  Stream_Valid/1 -> CtrlGen/2(Stream_Valid)
  Line Buffer/3 -> shftEnable/1
  Line Buffer/1 -> pixel/1

== system PE_V2_0/2DConvPE1 V2.0/MaxPooling/OutValidGen ==
  ctrl : Inport
  Window_Width : Inport  Port=2
  Feature_Height : Inport  Port=3
  Compare To Constant : simulink/Logic and Bit Operations/Compare To Constant  Commented=on  relop=>  const=0  OutDataTypeStr=boolean
  Constant : Constant  OutDataTypeStr=uint32  SampleTime=-1
  Delay36 : Delay  DelayLength=1
  Logical Operator1 : Logic  Operator=NOT  AllPortsSameDT=off  OutDataTypeStr=boolean
  Logical Operator3 : Logic  Inputs=3  AllPortsSameDT=off  OutDataTypeStr=boolean
  Logical Operator4 : Logic  Operator=NOT  AllPortsSameDT=off  OutDataTypeStr=boolean
  Logical Operator5 : Logic  Operator=OR  AllPortsSameDT=off  OutDataTypeStr=boolean
  Logical Operator6 : Logic  Operator=NOT  Inputs=3  AllPortsSameDT=off  OutDataTypeStr=boolean
  Minus1 : Sum  Inputs=+-
  Minus2 : Sum  Inputs=+-
  NumRow_Counter : hdlsllib/Sources/HDL Counter  CountType=Free running  CountInit=0  CountStep=1  CountMax=2^15  CountFromType=Initial value  CountFrom=0  CountResetPort=on  CountLoadPort=off  CountEnbPort=on  CountDirPort=off  CountDataType=Unsigned  CountWordLen=32  CountFracLen=0  CountSampTime=1
  Pixel Control Bus Selector : BusSelector  OutputSignals=hStart,hEnd,vStart,vEnd,valid
  Relational Operator1 : RelationalOperator  Operator=<  OutDataTypeStr=boolean  RndMeth=Nearest
  Relational Operator2 : RelationalOperator  Operator=<=  OutDataTypeStr=boolean  RndMeth=Nearest
  Row_Counter : hdlsllib/Sources/HDL Counter  CountType=Free running  CountInit=0  CountStep=1  CountMax=2^15  CountFromType=Initial value  CountFrom=0  CountResetPort=on  CountLoadPort=off  CountEnbPort=on  CountDirPort=off  CountDataType=Unsigned  CountWordLen=32  CountFracLen=0  CountSampTime=1
  Terminator1 : Terminator
  Out1 : Outport
  wires:
  NumRow_Counter/1 -> Relational Operator2/2, Compare To Constant/1
  Pixel Control Bus Selector/1 -> NumRow_Counter/2  "<hStart>"
  Minus2/1 -> Relational Operator2/1
  Relational Operator1/1 -> Logical Operator4/1
  Pixel Control Bus Selector/3 -> Logical Operator5/1  "<vStart>"
  Feature_Height/1 -> Minus2/1
  Minus1/1 -> Relational Operator1/2
  Row_Counter/1 -> Relational Operator1/1
  Pixel Control Bus Selector/5 -> Row_Counter/2, Logical Operator1/1, Logical Operator3/2  "<valid>"
  Window_Width/1 -> Minus1/1
  Pixel Control Bus Selector/2 -> Terminator1/1  "<hEnd>"
  Delay36/1 -> Pixel Control Bus Selector/1
  Constant/1 -> Minus1/2, Minus2/2
  Logical Operator6/1 -> Logical Operator3/1
  Logical Operator5/1 -> NumRow_Counter/1
  Pixel Control Bus Selector/4 -> Logical Operator5/2  "<vEnd>"
  Relational Operator2/1 -> Logical Operator6/1
  Logical Operator1/1 -> Row_Counter/1
  Logical Operator4/1 -> Logical Operator3/3
  Logical Operator3/1 -> Out1/1
  ctrl/1 -> Delay36/1

== system PE_V2_0/2DConvPE1 V2.0/MaxPooling/window Selector ==
  pixel : Inport
  valid : Inport  Port=2
  step : Inport  Port=3
  Add : Sum  Inputs=+-
  Compare To Zero : simulink/Logic and Bit Operations/Compare To Zero  relop===  OutDataTypeStr=boolean
  Constant : Constant  OutDataTypeStr=uint32
  Delay : Delay
  Delay1 : Delay  DelayLength=1
  Delay36 : Delay  DelayLength=1
  Logical Operator : Logic  Operator=NOT  AllPortsSameDT=off  OutDataTypeStr=boolean
  Logical Operator1 : Logic  Operator=OR  AllPortsSameDT=off  OutDataTypeStr=boolean
  Logical Operator2 : Logic  AllPortsSameDT=off  OutDataTypeStr=boolean
  Relational Operator : RelationalOperator  OutDataTypeStr=boolean  RndMeth=Nearest
  Selector1 : Selector  InputPortWidth=2  IndexOptions=Index vector (dialog)  Indices=[1]  OutputSizes=1
  Selector2 : Selector  InputPortWidth=2  IndexOptions=Index vector (dialog)  Indices=[2]  OutputSizes=1
  Selector3 : Selector  InputPortWidth=2  IndexOptions=Index vector (dialog)  Indices=[1]  OutputSizes=1
  Selector4 : Selector  InputPortWidth=2  IndexOptions=Index vector (dialog)  Indices=[2]  OutputSizes=1
  Step Counter : hdlsllib/Sources/HDL Counter  CountType=Free running  CountInit=0  CountStep=1  CountMax=2^15  CountFromType=Initial value  CountFrom=0  CountResetPort=on  CountLoadPort=off  CountEnbPort=on  CountDirPort=off  CountDataType=Unsigned  CountWordLen=32  CountFracLen=0  CountSampTime=1
  Out1 : Outport
  Out2 : Outport  Port=2
  Out3 : Outport  Port=3
  Out4 : Outport  Port=4
  Valid : Outport  Port=5
  wires:
  Selector2/1 -> Out2/1
  Delay/1 -> Selector4/1, Selector3/1
  Selector3/1 -> Out3/1
  Selector1/1 -> Out1/1
  Selector4/1 -> Out4/1
  pixel/1 -> Delay36/1, Delay/1
  Step Counter/1 -> Compare To Zero/1, Relational Operator/1
  Delay1/1 -> Logical Operator2/2, Step Counter/2, Logical Operator/1
  Logical Operator/1 -> Logical Operator1/2
  step/1 -> Add/1
  Constant/1 -> Add/2
  Add/1 -> Relational Operator/2
  Relational Operator/1 -> Logical Operator1/1
  Logical Operator1/1 -> Step Counter/1
  Compare To Zero/1 -> Logical Operator2/1
  Logical Operator2/1 -> Valid/1
  Delay36/1 -> Selector2/1, Selector1/1
  valid/1 -> Delay1/1

== system PE_V2_0/2DCov PEV1.1/Address Logic/  ==
  In1 : Inport
  In2 : Inport  Port=2
  Constant1 : Constant  Value=0  OutDataTypeStr=uint32
  Constant2 : Constant  Value=0  OutDataTypeStr=uint32
  Logical Operator3 : Logic  Operator=NOT  AllPortsSameDT=off  OutDataTypeStr=boolean
  Switch : Switch  Criteria=u2 ~= 0
  Switch1 : Switch  Criteria=u2 ~= 0
  addr_bit_sel1 : hdlsllib/Logic and Bit Operations/Bit Slice  lidx=12  ridx=0
  addr_bit_sel2 : hdlsllib/Logic and Bit Operations/Bit Slice  lidx=12  ridx=0
  W : Outport
  R : Outport  Port=2
  wires:
  In2/1 -> Switch/2, Logical Operator3/1
  Constant1/1 -> Switch/1
  Switch1/1 -> addr_bit_sel1/1
  In1/1 -> Switch1/3, Switch/3
  Logical Operator3/1 -> Switch1/2
  Constant2/1 -> Switch1/1
  Switch/1 -> addr_bit_sel2/1
  addr_bit_sel1/1 -> W/1  "vec_wr_addr"
  addr_bit_sel2/1 -> R/1  "vec_wr_addr"

== system PE_V2_0/2DCov PEV1.1/LIne Buffer/Line Buffer ==
  Stream_In : Inport
  Stream_Valid : Inport  Port=2
  Feature_Area : Inport  Port=3
  Feature_Width : Inport  Port=4
  CtrlGen : Subsystem
  Line Buffer : visionhdlutilities/Line Buffer  NeighborhoodSize=[3 1]  PaddingMethod=Constant  PaddingValue=0  LineBufferSize=128  SimulateUsing=Code generation
      settings: SourceProductBaseCode=VT
  pixel : Outport
  ctrl : Outport  Port=2
  shftEnable : Outport  Port=3
  wires:
  Feature_Area/1 -> CtrlGen/3(Feature_Area)
  Line Buffer/2 -> ctrl/1
  CtrlGen/1(StreamOut) -> Line Buffer/1
  Feature_Width/1 -> CtrlGen/4(Feature_Width)
  Stream_In/1 -> CtrlGen/1(Stream_In)
  CtrlGen/2(Ctrl) -> Line Buffer/2
  Stream_Valid/1 -> CtrlGen/2(Stream_Valid)
  Line Buffer/3 -> shftEnable/1
  Line Buffer/1 -> pixel/1

== system PE_V2_0/2DCov PEV1.1/LIne Buffer/OutValidGen ==
  In1 : Inport
  Weight_Width : Inport  Port=2
  Feature_Height : Inport  Port=3
  Compare To Constant : simulink/Logic and Bit Operations/Compare To Constant  relop=>  const=0  OutDataTypeStr=boolean
  Constant : Constant  OutDataTypeStr=uint32  SampleTime=-1
  Delay2 : Delay  DelayLength=1
  Logical Operator1 : Logic  Operator=NOT  AllPortsSameDT=off  OutDataTypeStr=boolean
  Logical Operator2 : Logic  Operator=OR  AllPortsSameDT=off  OutDataTypeStr=boolean
  Logical Operator3 : Logic  Inputs=4  AllPortsSameDT=off  OutDataTypeStr=boolean
  Logical Operator4 : Logic  Operator=NOT  AllPortsSameDT=off  OutDataTypeStr=boolean
  Logical Operator5 : Logic  Operator=OR  AllPortsSameDT=off  OutDataTypeStr=boolean
  Logical Operator6 : Logic  Operator=NOT  Inputs=3  AllPortsSameDT=off  OutDataTypeStr=boolean
  Minus1 : Sum  Inputs=+--
  Minus2 : Sum  Inputs=+-
  NumRow_Counter : hdlsllib/Sources/HDL Counter  CountType=Free running  CountInit=0  CountStep=1  CountMax=2^15  CountFromType=Initial value  CountFrom=0  CountResetPort=on  CountLoadPort=off  CountEnbPort=on  CountDirPort=off  CountDataType=Unsigned  CountWordLen=32  CountFracLen=0  CountSampTime=1
  Pixel Control Bus Selector : BusSelector  OutputSignals=hStart,hEnd,vStart,vEnd,valid
  Relational Operator1 : RelationalOperator  Operator=<  OutDataTypeStr=boolean  RndMeth=Nearest
  Relational Operator2 : RelationalOperator  Operator=<=  OutDataTypeStr=boolean  RndMeth=Nearest
  Row_Counter : hdlsllib/Sources/HDL Counter  CountType=Free running  CountInit=0  CountStep=1  CountMax=2^15  CountFromType=Initial value  CountFrom=0  CountResetPort=on  CountLoadPort=off  CountEnbPort=on  CountDirPort=off  CountDataType=Unsigned  CountWordLen=32  CountFracLen=0  CountSampTime=1
  Terminator1 : Terminator
  valid : Outport
  wires:
  Compare To Constant/1 -> Logical Operator3/2
  NumRow_Counter/1 -> Relational Operator2/2, Compare To Constant/1
  Pixel Control Bus Selector/1 -> NumRow_Counter/2, Logical Operator2/1  "<hStart>"
  Minus2/1 -> Relational Operator2/1
  Relational Operator1/1 -> Logical Operator4/1
  Logical Operator1/1 -> Logical Operator2/2
  Pixel Control Bus Selector/3 -> Logical Operator5/1  "<vStart>"
  Feature_Height/1 -> Minus2/1
  Minus1/1 -> Relational Operator1/2
  Row_Counter/1 -> Relational Operator1/1
  Pixel Control Bus Selector/5 -> Logical Operator1/1, Row_Counter/2, Logical Operator3/3  "<valid>"
  Weight_Width/1 -> Minus1/1
  Pixel Control Bus Selector/2 -> Terminator1/1  "<hEnd>"
  Delay2/1 -> Pixel Control Bus Selector/1
  Constant/1 -> Minus1/3, Minus1/2, Minus2/2
  Logical Operator6/1 -> Logical Operator3/1
  Logical Operator5/1 -> NumRow_Counter/1
  Pixel Control Bus Selector/4 -> Logical Operator5/2  "<vEnd>"
  Relational Operator2/1 -> Logical Operator6/1
  Logical Operator2/1 -> Row_Counter/1
  Logical Operator4/1 -> Logical Operator3/4
  Logical Operator3/1 -> valid/1
  In1/1 -> Delay2/1

== system PE_V2_0/2DCov PEV1.1/MaxPooling/Comparator ==
  In1 : Inport
  In2 : Inport  Port=2
  In3 : Inport  Port=3
  In4 : Inport  Port=4
  Valid : Inport  Port=5
  Delay{,1..4} (5 alike) : Delay  DelayLength=1
  Relational Operator : RelationalOperator  Operator=>  OutDataTypeStr=boolean  RndMeth=Nearest
  Relational Operator1 : RelationalOperator  Operator=>  OutDataTypeStr=boolean  RndMeth=Nearest
  Relational Operator2 : RelationalOperator  Operator=>  OutDataTypeStr=boolean  RndMeth=Nearest
  Switch : Switch  Criteria=u2 > Threshold
  Switch1 : Switch  Criteria=u2 > Threshold
  Switch2 : Switch  Criteria=u2 > Threshold
  Out1 : Outport
  outvalid : Outport  Port=2
  wires:
  Switch1/1 -> Relational Operator2/2, Switch2/3
  Switch/1 -> Switch2/1, Relational Operator2/1
  Delay/1 -> Switch/1, Relational Operator/1
  Relational Operator/1 -> Switch/2
  Relational Operator1/1 -> Switch1/2
  In2/1 -> Delay1/1
  In3/1 -> Delay2/1
  Relational Operator2/1 -> Switch2/2
  In4/1 -> Delay3/1
  Switch2/1 -> Out1/1
  Valid/1 -> Delay4/1
  Delay1/1 -> Relational Operator/2, Switch/3
  Delay2/1 -> Switch1/1, Relational Operator1/1
  In1/1 -> Delay/1
  Delay3/1 -> Relational Operator1/2, Switch1/3
  Delay4/1 -> outvalid/1

== system PE_V2_0/2DCov PEV1.1/MaxPooling/Line Buffer1 ==
  Stream_In : Inport
  Stream_Valid : Inport  Port=2
  Feature_Area : Inport  Port=3
  Feature_Width : Inport  Port=4
  CtrlGen : Subsystem
  Line Buffer : visionhdlutilities/Line Buffer  NeighborhoodSize=[2 1]  PaddingMethod=Constant  PaddingValue=0  LineBufferSize=128  SimulateUsing=Code generation
      settings: SourceProductBaseCode=VT
  pixel : Outport
  ctrl : Outport  Port=2
  shftEnable : Outport  Port=3
  wires:
  Feature_Area/1 -> CtrlGen/3(Feature_Area)
  Line Buffer/2 -> ctrl/1
  CtrlGen/1(StreamOut) -> Line Buffer/1
  Feature_Width/1 -> CtrlGen/4(Feature_Width)
  Stream_In/1 -> CtrlGen/1(Stream_In)
  CtrlGen/2(Ctrl) -> Line Buffer/2
  Stream_Valid/1 -> CtrlGen/2(Stream_Valid)
  Line Buffer/3 -> shftEnable/1
  Line Buffer/1 -> pixel/1
